simulink model "mymodel_v1"  (R2020b)
settings: Solver=FixedStepAuto  StartTime=0  StopTime=1  FixedStep=Ts  RelTol=1e-3
undefined symbols (not defined in the file or in its folder): Ts, Wbase
libraries: SimplusGT x8, powerlib x5
settings Model: Creator=admin_user  LastModifiedBy=admin_user

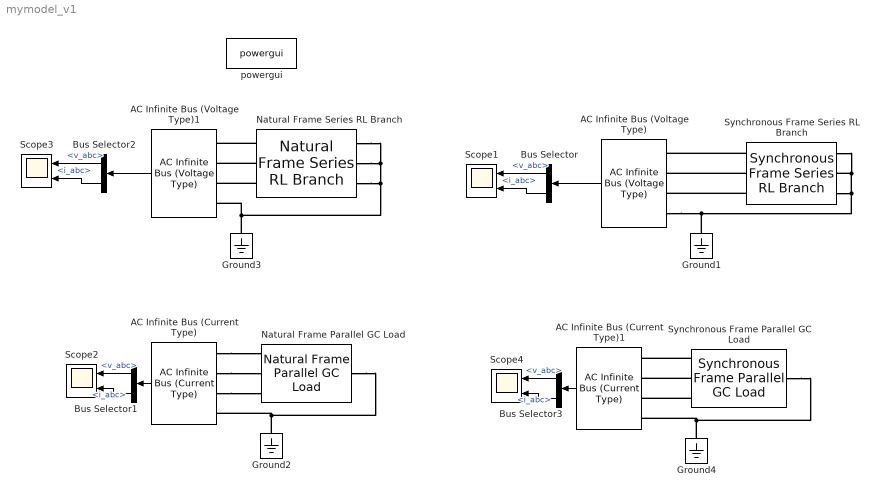
== system mymodel_v1 ==
  AC Infinite Bus (Current Type) : SimplusGT/AC Infinite Bus (Current Type)  Ts=Ts  Sbase=1  Vbase=1  Wbase=Wbase  id=1  iq=0  theta0=0  w=1  R=1e-9  C=1e-9
      settings: SourceProductName=Simplus Grid Tool
  AC Infinite Bus (Current Type)1 : SimplusGT/AC Infinite Bus (Current Type)  Ts=Ts  Sbase=1  Vbase=1  Wbase=Wbase  id=1  iq=0  theta0=0  w=1  R=1e-9  C=1e-9
      settings: SourceProductName=Simplus Grid Tool
  AC Infinite Bus (Voltage Type) : SimplusGT/AC Infinite Bus (Voltage Type)  Ts=Ts  Sbase=1  Vbase=1  Wbase=Wbase  vd=1  vq=0  theta0=0  w=Wbase  R=1e-30
      settings: SourceProductName=Simplus Grid Tool
  AC Infinite Bus (Voltage Type)1 : SimplusGT/AC Infinite Bus (Voltage Type)  Ts=Ts  Sbase=1  Vbase=1  Wbase=Wbase  vd=1  vq=0  theta0=0  w=Wbase  R=1e-30
      settings: SourceProductName=Simplus Grid Tool
  Bus Selector{,1..3} (4 alike) : BusSelector  OutputSignals=v_abc,i_abc
  Ground{1..4} (4 alike) : powerlib/Elements/Ground  LConnTagsString=a
  Natural Frame Parallel GC Load : SimplusGT/Natural Frame Parallel GC Load  Ts=Ts  G=0.1  C=1/Wbase
      settings: SourceProductName=Simplus Grid Tool
  Natural Frame Series RL Branch : SimplusGT/Natural Frame Series RL Branch  Ts=Ts  R=1e-2  L=1/Wbase
      settings: SourceProductName=Simplus Grid Tool
  Scope{1..4} (4 alike) : Scope  NumInputPorts=2
  Synchronous Frame Parallel GC Load : SimplusGT/Synchronous Frame Parallel GC Load  Ts=Ts  G=0.1  C=1/Wbase  w=Wbase
      settings: SourceProductName=Simplus Grid Tool
  Synchronous Frame Series RL Branch : SimplusGT/Synchronous Frame Series RL Branch  Ts=Ts  R=0.1  L=1/Wbase  w=Wbase
      settings: SourceProductName=Simplus Grid Tool
  powergui : powerlib/powergui  Priority=1  SimulationMode=Discrete  SampleTime=Ts  frequency=60  Iterations=50  frequencyindice=0  Pbase=100e6  ErrMax=1e-4  UnitsV=kV  UnitsW=MW  buscounter=0  FunctionMessages=off  echomessages=off  EnableUseOfTLC=off  CurrentSourceSwitches=off  DisableSnubberDevices=off  DisableRonSwitches=off  DisableVfSwitches=off  DisplayEquations=off  AutomaticDiscreteSolvers=off  SolverType=Tustin/Backward Euler (TBE)  Interpol=off  ExternalGateDelay=off  methode=off  Ts=100  x0status=blocks  SPID=on  SwTol=0  HookPort=off  NonlinearTolerance=1e-4  nMaxIteration=100  ContinueOnMaxIteration=off  RestoreLinks=warning  ResistiveCurrentMeasurement=off  Frange=[0:2:500]  Ylog=off  Xlog=on  ShowGrid=off  save=off  variable=ZData  structure=0  ZoomFFT=off  StartTime=0.0  cycles=1  DisplayStyle=1  fundamental=60  FreqAxis=off  MaxFrequency=1000  frequencyindicesteady=1  RmsSteady=1  display=off
  wires:
  AC Infinite Bus (Voltage Type)/1 -> Bus Selector/1
  Bus Selector/1 -> Scope1/1  "<v_abc>"
  Bus Selector/2 -> Scope1/2  "<i_abc>"
  AC Infinite Bus (Current Type)/1 -> Bus Selector1/1
  Bus Selector1/1 -> Scope2/1  "<v_abc>"
  Bus Selector1/2 -> Scope2/2  "<i_abc>"
  Bus Selector2/2 -> Scope3/2  "<i_abc>"
  AC Infinite Bus (Voltage Type)1/1 -> Bus Selector2/1
  Bus Selector2/1 -> Scope3/1  "<v_abc>"
  Bus Selector3/2 -> Scope4/2  "<i_abc>"
  AC Infinite Bus (Current Type)1/1 -> Bus Selector3/1
  Bus Selector3/1 -> Scope4/1  "<v_abc>"
  connections:
  Synchronous Frame Series RL Branch/LConn1 -- AC Infinite Bus (Voltage Type)/LConn1
  Synchronous Frame Series RL Branch/LConn2 -- AC Infinite Bus (Voltage Type)/LConn2
  Synchronous Frame Series RL Branch/LConn3 -- AC Infinite Bus (Voltage Type)/LConn3
  Synchronous Frame Series RL Branch/RConn1 -- Ground1/LConn1 -- AC Infinite Bus (Voltage Type)/LConn4 -- Synchronous Frame Series RL Branch/RConn3 -- Synchronous Frame Series RL Branch/RConn2
  Ground2/LConn1 -- Natural Frame Parallel GC Load/LConn1 -- AC Infinite Bus (Current Type)/LConn4
  AC Infinite Bus (Current Type)/LConn1 -- Natural Frame Parallel GC Load/RConn1
  AC Infinite Bus (Current Type)/LConn2 -- Natural Frame Parallel GC Load/RConn2
  AC Infinite Bus (Current Type)/LConn3 -- Natural Frame Parallel GC Load/RConn3
  Natural Frame Series RL Branch/LConn1 -- AC Infinite Bus (Voltage Type)1/LConn1
  Natural Frame Series RL Branch/LConn2 -- AC Infinite Bus (Voltage Type)1/LConn2
  Natural Frame Series RL Branch/LConn3 -- AC Infinite Bus (Voltage Type)1/LConn3
  Ground3/LConn1 -- Natural Frame Series RL Branch/RConn1 -- Natural Frame Series RL Branch/RConn2 -- Natural Frame Series RL Branch/RConn3 -- AC Infinite Bus (Voltage Type)1/LConn4
  Ground4/LConn1 -- Synchronous Frame Parallel GC Load/LConn1 -- AC Infinite Bus (Current Type)1/LConn4
  Synchronous Frame Parallel GC Load/RConn3 -- AC Infinite Bus (Current Type)1/LConn3
  Synchronous Frame Parallel GC Load/RConn1 -- AC Infinite Bus (Current Type)1/LConn1
  Synchronous Frame Parallel GC Load/RConn2 -- AC Infinite Bus (Current Type)1/LConn2
